simulink model "test14623_4"  (R2025b)
settings: Solver=VariableStepAuto  StartTime=0.0  StopTime=20  RelTol=1e-3
settings Model: Creator=jx2004  LastModifiedBy=jx2004

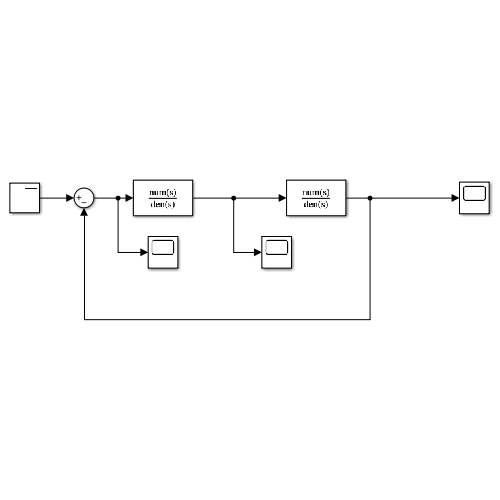
[thumbnail: Simulink's stored preview of the top-level diagram]
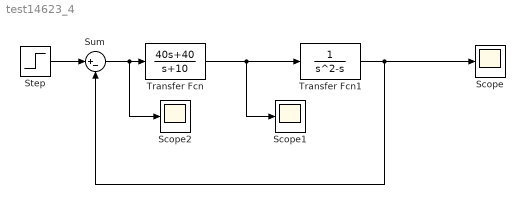
== system test14623_4 ==
  Scope : Scope
      settings: ActiveDisplayYMinimum=-0.19109667179195569  ActiveDisplayYMaximum=1.7198700461276017
  Scope1 : Scope
      settings: ActiveDisplayYMinimum=-16.385527748959646  ActiveDisplayYMaximum=46.2650586387733
  Scope2 : Scope
      settings: ActiveDisplayYMinimum=-0.71987004612760175  ActiveDisplayYMaximum=1.1910966717919558  DataLoggingVariableName=ScopeData2
  Step : Step  SampleTime=0
  Sum : Sum  Inputs=|+-
  Transfer Fcn : TransferFcn  Numerator=[40, 40]  Denominator=[1 10]
  Transfer Fcn1 : TransferFcn  Denominator=[1 -1 0]
  wires:
  Transfer Fcn/1 -> Scope1/1, Transfer Fcn1/1
  Transfer Fcn1/1 -> Scope/1, Sum/2
  Step/1 -> Sum/1
  Sum/1 -> Scope2/1, Transfer Fcn/1
